simulink model "w1p7_model"  (R2020a)
settings: Solver=VariableStepAuto  StartTime=0.0  StopTime=10.0  RelTol=1e-3
settings Model: Creator=avn19  LastModifiedBy=avn19

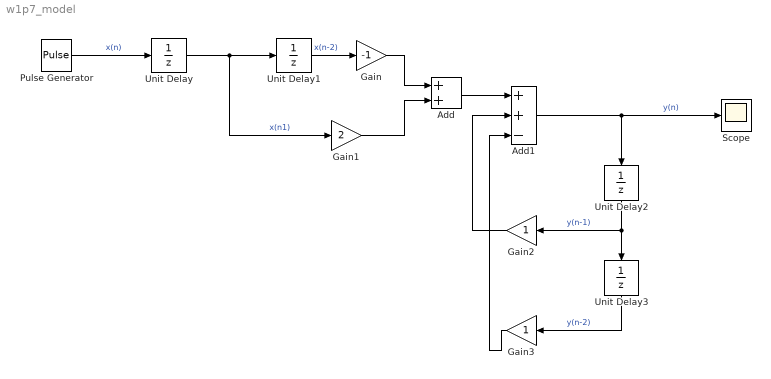
== system w1p7_model ==
  Add : Sum
  Add1 : Sum  Inputs=++-
  Gain : Gain  Gain=-1
  Gain1 : Gain  Gain=2
  Gain2 : Gain
  Gain3 : Gain
  Pulse Generator : DiscretePulseGenerator  PulseType=Time based  Period=10  PulseWidth=5
  Scope : Scope
  Unit Delay{,1..3} (4 alike) : UnitDelay  SampleTime=-1  HasFrameUpgradeWarning=on
  wires:
  Pulse Generator/1 -> Unit Delay/1  "x(n)"
  Unit Delay/1 -> Gain1/1, Unit Delay1/1  "x(n1)"
  Unit Delay1/1 -> Gain/1  "x(n-2)"
  Gain/1 -> Add/1
  Gain1/1 -> Add/2
  Add/1 -> Add1/1
  Add1/1 -> Unit Delay2/1, Scope/1  "y(n)"
  Unit Delay2/1 -> Gain2/1, Unit Delay3/1  "y(n-1)"
  Gain2/1 -> Add1/2
  Unit Delay3/1 -> Gain3/1  "y(n-2)"
  Gain3/1 -> Add1/3
